simulink model "general_pi_model"  (R2024b)
settings: Solver=VariableStepAuto  StartTime=0.0  StopTime=t_stop  RelTol=1e-3
values from neighbouring files (symbols this model uses):
  C = 1.97e3/2    (= 985)    [general_pi_init.m]
  L = 5.21e-5    (= 5.21e-05)    [general_pi_init.m]
  SIL = sqrt(L/C)    [general_pi_init.m]
libraries: fl_lib x128, nesl_utility x81, ee_lib x1
(part 1 of 3)
settings Model: Creator=inyongkim  LastModifiedBy=inyongkim

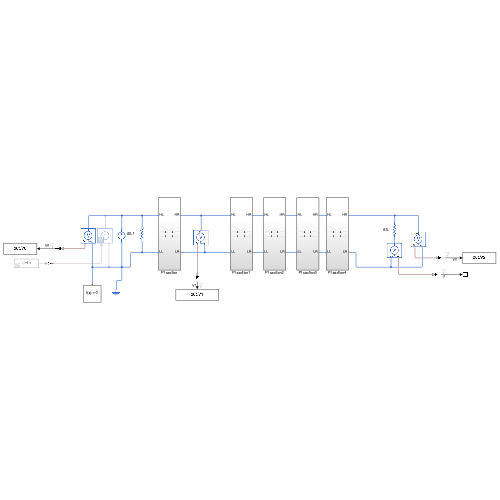
[thumbnail: Simulink's stored preview of the top-level diagram]
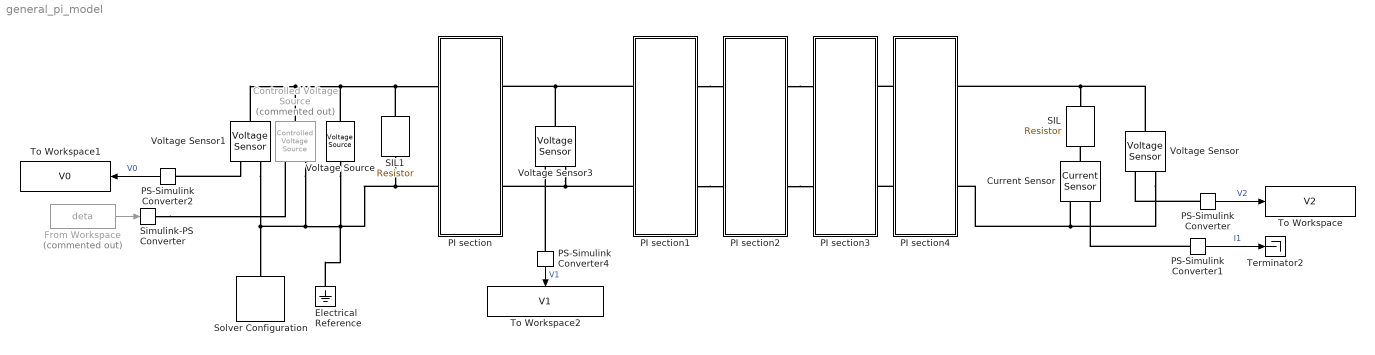
== system general_pi_model ==
  Controlled Voltage Source : fl_lib/Electrical/Electrical Sources/Controlled Voltage Source  Commented=on
  Current Sensor : fl_lib/Electrical/Electrical Sensors/Current Sensor
  Electrical Reference : fl_lib/Electrical/Electrical Elements/Electrical Reference
  From Workspace : FromWorkspace  Commented=on  VariableName=deta
  PI section : Subsystem
  PI section1 : Subsystem
  PI section2 : Subsystem
  PI section3 : Subsystem
  PI section4 : Subsystem
  PS-Simulink Converter{,1..2,4} (4 alike) : nesl_utility/PS-Simulink Converter  PhysicalDomain=network_engine_domain  SubClassName=ps_output  LeftPortType=input  RightPortType=output  PseudoPeriodic=off  Frequencies=[]  VectorFormat=inherit  Unit=inherit  AffineConversion=off
  SIL : fl_lib/Electrical/Electrical Elements/Resistor  R=SIL Ohm  i_specify=off  i_priority=None  i=0 A  i_nominal_specify=off  i_nominal_value=1  i_nominal_unit=A  v_specify=off  v_priority=None  v=0 V  v_nominal_specify=off  v_nominal_value=1  v_nominal_unit=V
  SIL1 : fl_lib/Electrical/Electrical Elements/Resistor  R=SIL*1e12 Ohm  i_specify=off  i_priority=None  i=0 A  i_nominal_specify=off  i_nominal_value=1  i_nominal_unit=A  v_specify=off  v_priority=None  v=0 V  v_nominal_specify=off  v_nominal_value=1  v_nominal_unit=V
  Simulink-PS Converter : nesl_utility/Simulink-PS Converter  PhysicalDomain=network_engine_domain  SubClassName=ps_input  LeftPortType=input  RightPortType=output  PseudoPeriodic=off  Frequencies=[]  NoiseDistribution=none  NoiseParameters=[]  Unit=V  AffineConversion=off  FilteringAndDerivatives=provide  SimscapeFilterOrder=1  InputFilterTimeConstant=0.001  UdotUserProvided=0
  Solver Configuration : nesl_utility/Solver Configuration  PhysicalDomain=network_engine_domain  SubClassName=solver  LeftPortType=input  RightPortType=generic  Tones=[]  Harmonics=[]  SimulateNoise=off  Profile=off  UseLocalSampling=off  EnableSwitchedLinearOptims=on  FrequencyDomain=off  UseCCode=off  RelTol=0.001  AbsTol=0.001  MinStep=1e-09  ToWorkspace=off  RevertToSquareIcSolve=off  NumHomotopyIterations=100  PhasorMode=off  PhasorModeNumHarmonics=1  ConsistencySolver=NEWTON_XTOL_AFTER_FTOL  IndexReductionMethod=DerivativeReplacement  DoDC=off  ResidualTolerance=1e-09  ConsistencyTolSource=GLOBAL  ConsistencyAbsTol=0.001  ConsistencyRelTol=0.001  ConsistencyTolFactor=0.001  UseLocalSolver=off  LocalSolverChoice=NE_BACKWARD_EULER_ADVANCER  ResolveIndetEquations=on  FunctionEvalNumThread=1  LocalSolverSampleTime=0.001  DoFixedCost=off  MaxNonlinIter=3  MaxModeIter=2  ComputeImpulses=off  ImpulseIterations=2  LinearAlgebra=auto  LinearAlgebraNumThread=0  EquationFormulation=NE_TIME_EF  DelaysMemoryBudget=1024  AutomaticFiltering=on  FilteringTimeConstant=0.001  PartitionStorageMethod=AS_NEEDED  PartitionMemoryBudget=1024  PartitionMethod=ROBUST  MultibodyUseLocalSolver=off  MultibodyLocalSolverChoice=ODE1  MultibodyLocalSolverSampleTime=0.001
  Terminator2 : Terminator
  To Workspace : ToWorkspace  VariableName=V2  SaveFormat=Timeseries  SampleTime=-1
  To Workspace1 : ToWorkspace  VariableName=V0  SaveFormat=Timeseries  SampleTime=-1
  To Workspace2 : ToWorkspace  VariableName=V1  SaveFormat=Timeseries  SampleTime=-1
  Voltage Sensor : fl_lib/Electrical/Electrical Sensors/Voltage Sensor
  Voltage Sensor1 : fl_lib/Electrical/Electrical Sensors/Voltage Sensor
  Voltage Sensor3 : fl_lib/Electrical/Electrical Sensors/Voltage Sensor
  Voltage Source : ee_lib/Sources/Voltage Source  dc_voltage=0 V  ac_voltage=1 V  ac_shift=0 rad  ac_frequency=0.1 Hz  noise_mode=ee.enum.sources.noise.Disabled  PSD=0 V^2/Hz  sample_time=1e-3 s  repeatability=ee.enum.sources.repeatability.NotRepeatable  user_seed=0  auto_seed=3499211588  i_specify=off  i_priority=None  i=0 A  i_nominal_specify=off  i_nominal_value=1  i_nominal_unit=A  v_specify=off  v_priority=None  v=0 V  v_nominal_specify=off  v_nominal_value=1  v_nominal_unit=V
  wires:
  PS-Simulink Converter/1 -> To Workspace/1  "V2"
  PS-Simulink Converter1/1 -> Terminator2/1  "I1"
  PS-Simulink Converter2/1 -> To Workspace1/1  "V0"
  From Workspace/1 -> Simulink-PS Converter/1
  PS-Simulink Converter4/1 -> To Workspace2/1  "V1"
  connections:
  Voltage Source/RConn1 -- Controlled Voltage Source/RConn2 -- Solver Configuration/RConn1 -- Voltage Sensor1/RConn2 -- SIL1/RConn1 -- PI section/LConn2 -- Electrical Reference/LConn1
  Voltage Sensor1/LConn1 -- SIL1/LConn1 -- PI section/LConn1 -- Voltage Source/LConn1 -- Controlled Voltage Source/LConn1
  Voltage Sensor/LConn1 -- PI section4/RConn1 -- SIL/LConn1
  PS-Simulink Converter/LConn1 -- Voltage Sensor/RConn1
  Current Sensor/LConn1 -- SIL/RConn1
  PS-Simulink Converter1/LConn1 -- Current Sensor/RConn1
  Voltage Sensor1/RConn1 -- PS-Simulink Converter2/LConn1
  Simulink-PS Converter/RConn1 -- Controlled Voltage Source/RConn1
  PS-Simulink Converter4/LConn1 -- Voltage Sensor3/RConn1
  Voltage Sensor3/LConn1 -- PI section1/LConn1 -- PI section/RConn1
  Voltage Sensor3/RConn2 -- PI section/RConn2 -- PI section1/LConn2
  Voltage Sensor/RConn2 -- PI section4/RConn2 -- Current Sensor/RConn2
  PI section1/RConn1 -- PI section2/LConn1
  PI section1/RConn2 -- PI section2/LConn2
  PI section2/RConn1 -- PI section3/LConn1
  PI section2/RConn2 -- PI section3/LConn2
  PI section4/LConn1 -- PI section3/RConn1
  PI section4/LConn2 -- PI section3/RConn2

== system general_pi_model/PI section ==
  General C : Subsystem
      settings: PortSchema="{\"entries\":[{\"content\":{\"sides\":[{\"content\":{},\"type\":\"ConnectorPlacement.EquallySpacedRectSide\",\"uuid\":\"54c7c027-76dd-4589-a14d-62021aaba10d\"},{\"content\":{\"side\":\"RIGHT\"},\"type\":\"ConnectorPlacement.EquallySpacedRectSide\",\"uuid\":\"5fae45fc-fbd0-44d0-9d3d-94b3e56c48e3\"},{\"content\":{\"connectorIds\":[\"LConn1\"],\"side\":\"TOP\"},\"type\":\"ConnectorPlacement.EquallySpacedRectSide\",\"uuid\":\"b6847d7e-9825-46ad-84aa-5df9156d119d\"},{\"content\":{\"connectorIds\":[\"RConn1\"],\"side\":\"BOTTOM\"},\"type\":\"ConnectorPlacement.EquallySpacedRectSide\",\"uuid\":\"1394d42d-8985-4309-a3e0-31ed6b8c9496\"}]},\"type\":\"ConnectorPlacement.EquallySpacedConnector\",\"uuid\":\"6a4af355-2598-47af-9220-e6e09375ad72\"}],\"packageUris\":[\"http://schema.mathworks.com/mf0/Connector/R2020b\"],\"version\":\"1.0\"}"
  General C1 : Subsystem
      settings: PortSchema="{\"entries\":[{\"content\":{\"sides\":[{\"content\":{},\"type\":\"ConnectorPlacement.EquallySpacedRectSide\",\"uuid\":\"54c7c027-76dd-4589-a14d-62021aaba10d\"},{\"content\":{\"side\":\"RIGHT\"},\"type\":\"ConnectorPlacement.EquallySpacedRectSide\",\"uuid\":\"5fae45fc-fbd0-44d0-9d3d-94b3e56c48e3\"},{\"content\":{\"connectorIds\":[\"LConn1\"],\"side\":\"TOP\"},\"type\":\"ConnectorPlacement.EquallySpacedRectSide\",\"uuid\":\"b6847d7e-9825-46ad-84aa-5df9156d119d\"},{\"content\":{\"connectorIds\":[\"RConn1\"],\"side\":\"BOTTOM\"},\"type\":\"ConnectorPlacement.EquallySpacedRectSide\",\"uuid\":\"1394d42d-8985-4309-a3e0-31ed6b8c9496\"}]},\"type\":\"ConnectorPlacement.EquallySpacedConnector\",\"uuid\":\"6a4af355-2598-47af-9220-e6e09375ad72\"}],\"packageUris\":[\"http://schema.mathworks.com/mf0/Connector/R2020b\"],\"version\":\"1.0\"}"
  General L : Subsystem
      settings: PortSchema="{\"entries\":[{\"content\":{\"sides\":[{\"content\":{},\"type\":\"ConnectorPlacement.EquallySpacedRectSide\",\"uuid\":\"54c7c027-76dd-4589-a14d-62021aaba10d\"},{\"content\":{\"side\":\"RIGHT\"},\"type\":\"ConnectorPlacement.EquallySpacedRectSide\",\"uuid\":\"5fae45fc-fbd0-44d0-9d3d-94b3e56c48e3\"},{\"content\":{\"connectorIds\":[\"LConn1\"],\"side\":\"TOP\"},\"type\":\"ConnectorPlacement.EquallySpacedRectSide\",\"uuid\":\"b6847d7e-9825-46ad-84aa-5df9156d119d\"},{\"content\":{\"connectorIds\":[\"RConn1\"],\"side\":\"BOTTOM\"},\"type\":\"ConnectorPlacement.EquallySpacedRectSide\",\"uuid\":\"7b301271-0a77-4acb-8843-591cb23b0585\"}]},\"type\":\"ConnectorPlacement.EquallySpacedConnector\",\"uuid\":\"6a4af355-2598-47af-9220-e6e09375ad72\"}],\"packageUris\":[\"http://schema.mathworks.com/mf0/Connector/R2020b\"],\"version\":\"1.0\"}"
  HL : PMIOPort  Side=Left
  HR : PMIOPort  Port=2  Side=Right
  LL : PMIOPort  Port=3  Side=Left
  LR : PMIOPort  Port=4  Side=Right
  connections:
  General L/RConn1 -- HR/RConn1 -- General C1/LConn1
  General C1/RConn1 -- General C/RConn1 -- LL/RConn1 -- LR/RConn1
  General C/LConn1 -- HL/RConn1 -- General L/LConn1

== system general_pi_model/PI section1 ==
  General C : Subsystem
      settings: PortSchema="{\"entries\":[{\"content\":{\"sides\":[{\"content\":{},\"type\":\"ConnectorPlacement.EquallySpacedRectSide\",\"uuid\":\"54c7c027-76dd-4589-a14d-62021aaba10d\"},{\"content\":{\"side\":\"RIGHT\"},\"type\":\"ConnectorPlacement.EquallySpacedRectSide\",\"uuid\":\"5fae45fc-fbd0-44d0-9d3d-94b3e56c48e3\"},{\"content\":{\"connectorIds\":[\"LConn1\"],\"side\":\"TOP\"},\"type\":\"ConnectorPlacement.EquallySpacedRectSide\",\"uuid\":\"b6847d7e-9825-46ad-84aa-5df9156d119d\"},{\"content\":{\"connectorIds\":[\"RConn1\"],\"side\":\"BOTTOM\"},\"type\":\"ConnectorPlacement.EquallySpacedRectSide\",\"uuid\":\"1394d42d-8985-4309-a3e0-31ed6b8c9496\"}]},\"type\":\"ConnectorPlacement.EquallySpacedConnector\",\"uuid\":\"6a4af355-2598-47af-9220-e6e09375ad72\"}],\"packageUris\":[\"http://schema.mathworks.com/mf0/Connector/R2020b\"],\"version\":\"1.0\"}"
  General C1 : Subsystem
      settings: PortSchema="{\"entries\":[{\"content\":{\"sides\":[{\"content\":{},\"type\":\"ConnectorPlacement.EquallySpacedRectSide\",\"uuid\":\"54c7c027-76dd-4589-a14d-62021aaba10d\"},{\"content\":{\"side\":\"RIGHT\"},\"type\":\"ConnectorPlacement.EquallySpacedRectSide\",\"uuid\":\"5fae45fc-fbd0-44d0-9d3d-94b3e56c48e3\"},{\"content\":{\"connectorIds\":[\"LConn1\"],\"side\":\"TOP\"},\"type\":\"ConnectorPlacement.EquallySpacedRectSide\",\"uuid\":\"b6847d7e-9825-46ad-84aa-5df9156d119d\"},{\"content\":{\"connectorIds\":[\"RConn1\"],\"side\":\"BOTTOM\"},\"type\":\"ConnectorPlacement.EquallySpacedRectSide\",\"uuid\":\"1394d42d-8985-4309-a3e0-31ed6b8c9496\"}]},\"type\":\"ConnectorPlacement.EquallySpacedConnector\",\"uuid\":\"6a4af355-2598-47af-9220-e6e09375ad72\"}],\"packageUris\":[\"http://schema.mathworks.com/mf0/Connector/R2020b\"],\"version\":\"1.0\"}"
  General L : Subsystem
      settings: PortSchema="{\"entries\":[{\"content\":{\"sides\":[{\"content\":{},\"type\":\"ConnectorPlacement.EquallySpacedRectSide\",\"uuid\":\"54c7c027-76dd-4589-a14d-62021aaba10d\"},{\"content\":{\"side\":\"RIGHT\"},\"type\":\"ConnectorPlacement.EquallySpacedRectSide\",\"uuid\":\"5fae45fc-fbd0-44d0-9d3d-94b3e56c48e3\"},{\"content\":{\"connectorIds\":[\"LConn1\"],\"side\":\"TOP\"},\"type\":\"ConnectorPlacement.EquallySpacedRectSide\",\"uuid\":\"b6847d7e-9825-46ad-84aa-5df9156d119d\"},{\"content\":{\"connectorIds\":[\"RConn1\"],\"side\":\"BOTTOM\"},\"type\":\"ConnectorPlacement.EquallySpacedRectSide\",\"uuid\":\"7b301271-0a77-4acb-8843-591cb23b0585\"}]},\"type\":\"ConnectorPlacement.EquallySpacedConnector\",\"uuid\":\"6a4af355-2598-47af-9220-e6e09375ad72\"}],\"packageUris\":[\"http://schema.mathworks.com/mf0/Connector/R2020b\"],\"version\":\"1.0\"}"
  HL : PMIOPort  Side=Left
  HR : PMIOPort  Port=2  Side=Right
  LL : PMIOPort  Port=3  Side=Left
  LR : PMIOPort  Port=4  Side=Right
  connections:
  General L/RConn1 -- General C1/LConn1 -- HR/RConn1
  LR/RConn1 -- General C1/RConn1 -- LL/RConn1 -- General C/RConn1
  General C/LConn1 -- General L/LConn1 -- HL/RConn1

== system general_pi_model/PI section2 ==
  General C : Subsystem
      settings: PortSchema="{\"entries\":[{\"content\":{\"sides\":[{\"content\":{},\"type\":\"ConnectorPlacement.EquallySpacedRectSide\",\"uuid\":\"54c7c027-76dd-4589-a14d-62021aaba10d\"},{\"content\":{\"side\":\"RIGHT\"},\"type\":\"ConnectorPlacement.EquallySpacedRectSide\",\"uuid\":\"5fae45fc-fbd0-44d0-9d3d-94b3e56c48e3\"},{\"content\":{\"connectorIds\":[\"LConn1\"],\"side\":\"TOP\"},\"type\":\"ConnectorPlacement.EquallySpacedRectSide\",\"uuid\":\"b6847d7e-9825-46ad-84aa-5df9156d119d\"},{\"content\":{\"connectorIds\":[\"RConn1\"],\"side\":\"BOTTOM\"},\"type\":\"ConnectorPlacement.EquallySpacedRectSide\",\"uuid\":\"1394d42d-8985-4309-a3e0-31ed6b8c9496\"}]},\"type\":\"ConnectorPlacement.EquallySpacedConnector\",\"uuid\":\"6a4af355-2598-47af-9220-e6e09375ad72\"}],\"packageUris\":[\"http://schema.mathworks.com/mf0/Connector/R2020b\"],\"version\":\"1.0\"}"
  General C1 : Subsystem
      settings: PortSchema="{\"entries\":[{\"content\":{\"sides\":[{\"content\":{},\"type\":\"ConnectorPlacement.EquallySpacedRectSide\",\"uuid\":\"54c7c027-76dd-4589-a14d-62021aaba10d\"},{\"content\":{\"side\":\"RIGHT\"},\"type\":\"ConnectorPlacement.EquallySpacedRectSide\",\"uuid\":\"5fae45fc-fbd0-44d0-9d3d-94b3e56c48e3\"},{\"content\":{\"connectorIds\":[\"LConn1\"],\"side\":\"TOP\"},\"type\":\"ConnectorPlacement.EquallySpacedRectSide\",\"uuid\":\"b6847d7e-9825-46ad-84aa-5df9156d119d\"},{\"content\":{\"connectorIds\":[\"RConn1\"],\"side\":\"BOTTOM\"},\"type\":\"ConnectorPlacement.EquallySpacedRectSide\",\"uuid\":\"1394d42d-8985-4309-a3e0-31ed6b8c9496\"}]},\"type\":\"ConnectorPlacement.EquallySpacedConnector\",\"uuid\":\"6a4af355-2598-47af-9220-e6e09375ad72\"}],\"packageUris\":[\"http://schema.mathworks.com/mf0/Connector/R2020b\"],\"version\":\"1.0\"}"
  General L : Subsystem
      settings: PortSchema="{\"entries\":[{\"content\":{\"sides\":[{\"content\":{},\"type\":\"ConnectorPlacement.EquallySpacedRectSide\",\"uuid\":\"54c7c027-76dd-4589-a14d-62021aaba10d\"},{\"content\":{\"side\":\"RIGHT\"},\"type\":\"ConnectorPlacement.EquallySpacedRectSide\",\"uuid\":\"5fae45fc-fbd0-44d0-9d3d-94b3e56c48e3\"},{\"content\":{\"connectorIds\":[\"LConn1\"],\"side\":\"TOP\"},\"type\":\"ConnectorPlacement.EquallySpacedRectSide\",\"uuid\":\"b6847d7e-9825-46ad-84aa-5df9156d119d\"},{\"content\":{\"connectorIds\":[\"RConn1\"],\"side\":\"BOTTOM\"},\"type\":\"ConnectorPlacement.EquallySpacedRectSide\",\"uuid\":\"7b301271-0a77-4acb-8843-591cb23b0585\"}]},\"type\":\"ConnectorPlacement.EquallySpacedConnector\",\"uuid\":\"6a4af355-2598-47af-9220-e6e09375ad72\"}],\"packageUris\":[\"http://schema.mathworks.com/mf0/Connector/R2020b\"],\"version\":\"1.0\"}"
  HL : PMIOPort  Side=Left
  HR : PMIOPort  Port=2  Side=Right
  LL : PMIOPort  Port=3  Side=Left
  LR : PMIOPort  Port=4  Side=Right
  connections:
  General L/RConn1 -- General C1/LConn1 -- HR/RConn1
  LR/RConn1 -- General C1/RConn1 -- LL/RConn1 -- General C/RConn1
  General C/LConn1 -- General L/LConn1 -- HL/RConn1

== system general_pi_model/PI section3 ==
  General C : Subsystem
      settings: PortSchema="{\"entries\":[{\"content\":{\"sides\":[{\"content\":{},\"type\":\"ConnectorPlacement.EquallySpacedRectSide\",\"uuid\":\"54c7c027-76dd-4589-a14d-62021aaba10d\"},{\"content\":{\"side\":\"RIGHT\"},\"type\":\"ConnectorPlacement.EquallySpacedRectSide\",\"uuid\":\"5fae45fc-fbd0-44d0-9d3d-94b3e56c48e3\"},{\"content\":{\"connectorIds\":[\"LConn1\"],\"side\":\"TOP\"},\"type\":\"ConnectorPlacement.EquallySpacedRectSide\",\"uuid\":\"b6847d7e-9825-46ad-84aa-5df9156d119d\"},{\"content\":{\"connectorIds\":[\"RConn1\"],\"side\":\"BOTTOM\"},\"type\":\"ConnectorPlacement.EquallySpacedRectSide\",\"uuid\":\"1394d42d-8985-4309-a3e0-31ed6b8c9496\"}]},\"type\":\"ConnectorPlacement.EquallySpacedConnector\",\"uuid\":\"6a4af355-2598-47af-9220-e6e09375ad72\"}],\"packageUris\":[\"http://schema.mathworks.com/mf0/Connector/R2020b\"],\"version\":\"1.0\"}"
  General C1 : Subsystem
      settings: PortSchema="{\"entries\":[{\"content\":{\"sides\":[{\"content\":{},\"type\":\"ConnectorPlacement.EquallySpacedRectSide\",\"uuid\":\"54c7c027-76dd-4589-a14d-62021aaba10d\"},{\"content\":{\"side\":\"RIGHT\"},\"type\":\"ConnectorPlacement.EquallySpacedRectSide\",\"uuid\":\"5fae45fc-fbd0-44d0-9d3d-94b3e56c48e3\"},{\"content\":{\"connectorIds\":[\"LConn1\"],\"side\":\"TOP\"},\"type\":\"ConnectorPlacement.EquallySpacedRectSide\",\"uuid\":\"b6847d7e-9825-46ad-84aa-5df9156d119d\"},{\"content\":{\"connectorIds\":[\"RConn1\"],\"side\":\"BOTTOM\"},\"type\":\"ConnectorPlacement.EquallySpacedRectSide\",\"uuid\":\"1394d42d-8985-4309-a3e0-31ed6b8c9496\"}]},\"type\":\"ConnectorPlacement.EquallySpacedConnector\",\"uuid\":\"6a4af355-2598-47af-9220-e6e09375ad72\"}],\"packageUris\":[\"http://schema.mathworks.com/mf0/Connector/R2020b\"],\"version\":\"1.0\"}"
  General L : Subsystem
      settings: PortSchema="{\"entries\":[{\"content\":{\"sides\":[{\"content\":{},\"type\":\"ConnectorPlacement.EquallySpacedRectSide\",\"uuid\":\"54c7c027-76dd-4589-a14d-62021aaba10d\"},{\"content\":{\"side\":\"RIGHT\"},\"type\":\"ConnectorPlacement.EquallySpacedRectSide\",\"uuid\":\"5fae45fc-fbd0-44d0-9d3d-94b3e56c48e3\"},{\"content\":{\"connectorIds\":[\"LConn1\"],\"side\":\"TOP\"},\"type\":\"ConnectorPlacement.EquallySpacedRectSide\",\"uuid\":\"b6847d7e-9825-46ad-84aa-5df9156d119d\"},{\"content\":{\"connectorIds\":[\"RConn1\"],\"side\":\"BOTTOM\"},\"type\":\"ConnectorPlacement.EquallySpacedRectSide\",\"uuid\":\"7b301271-0a77-4acb-8843-591cb23b0585\"}]},\"type\":\"ConnectorPlacement.EquallySpacedConnector\",\"uuid\":\"6a4af355-2598-47af-9220-e6e09375ad72\"}],\"packageUris\":[\"http://schema.mathworks.com/mf0/Connector/R2020b\"],\"version\":\"1.0\"}"
  HL : PMIOPort  Side=Left
  HR : PMIOPort  Port=2  Side=Right
  LL : PMIOPort  Port=3  Side=Left
  LR : PMIOPort  Port=4  Side=Right
  connections:
  General L/RConn1 -- General C1/LConn1 -- HR/RConn1
  LR/RConn1 -- General C1/RConn1 -- LL/RConn1 -- General C/RConn1
  General C/LConn1 -- General L/LConn1 -- HL/RConn1

== system general_pi_model/PI section4 ==
  General C : Subsystem
      settings: PortSchema="{\"entries\":[{\"content\":{\"sides\":[{\"content\":{},\"type\":\"ConnectorPlacement.EquallySpacedRectSide\",\"uuid\":\"54c7c027-76dd-4589-a14d-62021aaba10d\"},{\"content\":{\"side\":\"RIGHT\"},\"type\":\"ConnectorPlacement.EquallySpacedRectSide\",\"uuid\":\"5fae45fc-fbd0-44d0-9d3d-94b3e56c48e3\"},{\"content\":{\"connectorIds\":[\"LConn1\"],\"side\":\"TOP\"},\"type\":\"ConnectorPlacement.EquallySpacedRectSide\",\"uuid\":\"b6847d7e-9825-46ad-84aa-5df9156d119d\"},{\"content\":{\"connectorIds\":[\"RConn1\"],\"side\":\"BOTTOM\"},\"type\":\"ConnectorPlacement.EquallySpacedRectSide\",\"uuid\":\"1394d42d-8985-4309-a3e0-31ed6b8c9496\"}]},\"type\":\"ConnectorPlacement.EquallySpacedConnector\",\"uuid\":\"6a4af355-2598-47af-9220-e6e09375ad72\"}],\"packageUris\":[\"http://schema.mathworks.com/mf0/Connector/R2020b\"],\"version\":\"1.0\"}"
  General C1 : Subsystem
      settings: PortSchema="{\"entries\":[{\"content\":{\"sides\":[{\"content\":{},\"type\":\"ConnectorPlacement.EquallySpacedRectSide\",\"uuid\":\"54c7c027-76dd-4589-a14d-62021aaba10d\"},{\"content\":{\"side\":\"RIGHT\"},\"type\":\"ConnectorPlacement.EquallySpacedRectSide\",\"uuid\":\"5fae45fc-fbd0-44d0-9d3d-94b3e56c48e3\"},{\"content\":{\"connectorIds\":[\"LConn1\"],\"side\":\"TOP\"},\"type\":\"ConnectorPlacement.EquallySpacedRectSide\",\"uuid\":\"b6847d7e-9825-46ad-84aa-5df9156d119d\"},{\"content\":{\"connectorIds\":[\"RConn1\"],\"side\":\"BOTTOM\"},\"type\":\"ConnectorPlacement.EquallySpacedRectSide\",\"uuid\":\"1394d42d-8985-4309-a3e0-31ed6b8c9496\"}]},\"type\":\"ConnectorPlacement.EquallySpacedConnector\",\"uuid\":\"6a4af355-2598-47af-9220-e6e09375ad72\"}],\"packageUris\":[\"http://schema.mathworks.com/mf0/Connector/R2020b\"],\"version\":\"1.0\"}"
  General L : Subsystem
      settings: PortSchema="{\"entries\":[{\"content\":{\"sides\":[{\"content\":{},\"type\":\"ConnectorPlacement.EquallySpacedRectSide\",\"uuid\":\"54c7c027-76dd-4589-a14d-62021aaba10d\"},{\"content\":{\"side\":\"RIGHT\"},\"type\":\"ConnectorPlacement.EquallySpacedRectSide\",\"uuid\":\"5fae45fc-fbd0-44d0-9d3d-94b3e56c48e3\"},{\"content\":{\"connectorIds\":[\"LConn1\"],\"side\":\"TOP\"},\"type\":\"ConnectorPlacement.EquallySpacedRectSide\",\"uuid\":\"b6847d7e-9825-46ad-84aa-5df9156d119d\"},{\"content\":{\"connectorIds\":[\"RConn1\"],\"side\":\"BOTTOM\"},\"type\":\"ConnectorPlacement.EquallySpacedRectSide\",\"uuid\":\"7b301271-0a77-4acb-8843-591cb23b0585\"}]},\"type\":\"ConnectorPlacement.EquallySpacedConnector\",\"uuid\":\"6a4af355-2598-47af-9220-e6e09375ad72\"}],\"packageUris\":[\"http://schema.mathworks.com/mf0/Connector/R2020b\"],\"version\":\"1.0\"}"
  HL : PMIOPort  Side=Left
  HR : PMIOPort  Port=2  Side=Right
  LL : PMIOPort  Port=3  Side=Left
  LR : PMIOPort  Port=4  Side=Right
  connections:
  General L/RConn1 -- General C1/LConn1 -- HR/RConn1
  LR/RConn1 -- General C1/RConn1 -- LL/RConn1 -- General C/RConn1
  General C/LConn1 -- General L/LConn1 -- HL/RConn1

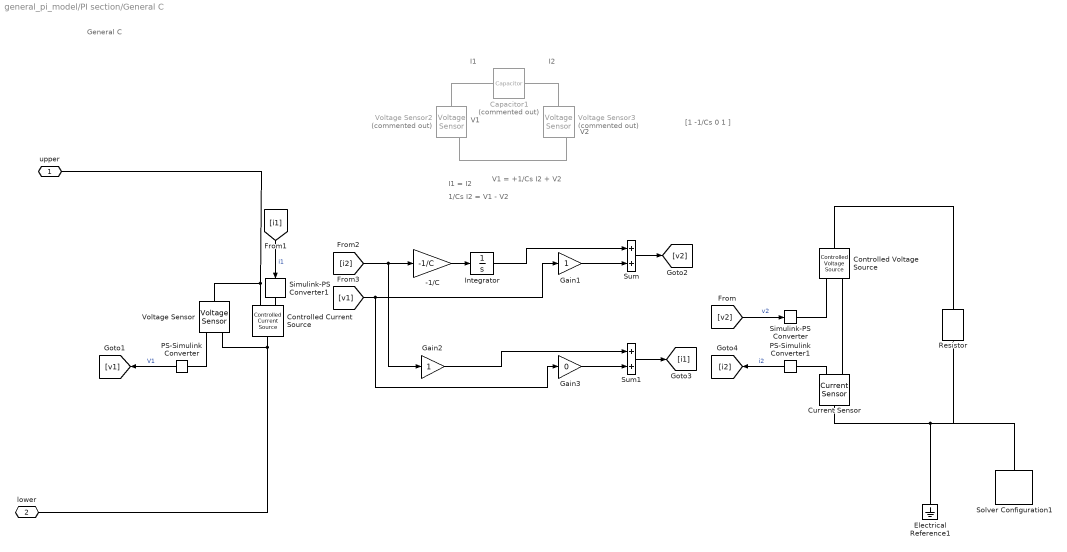
== system general_pi_model/PI section/General C ==
  note: General C
  note: V1
  note: V1 = +1/Cs I2 + V2
  note: I2
  note: I1 = I2
  note: 1/Cs I2 = V1 - V2
  note: V2
  note: [1 -1/Cs
      | 0 1 ]
  note: I1
  -1/C : Gain  Gain=-1/C
  Capacitor1 : fl_lib/Electrical/Electrical Elements/Capacitor  Commented=on  c=1e-6 F  r=1e-6 Ohm  g=0 1/Ohm  i_specify=off  i_priority=None  i=0 A  i_nominal_specify=off  i_nominal_value=1  i_nominal_unit=A  v_specify=off  v_priority=None  v=0 V  v_nominal_specify=off  v_nominal_value=1  v_nominal_unit=V  vc_specify=off  vc_priority=High  vc=0 V  vc_nominal_specify=off  vc_nominal_value=1  vc_nominal_unit=V
  Controlled Current Source : fl_lib/Electrical/Electrical Sources/Controlled Current Source
  Controlled Voltage Source : fl_lib/Electrical/Electrical Sources/Controlled Voltage Source
  Current Sensor : fl_lib/Electrical/Electrical Sensors/Current Sensor
  Electrical Reference1 : fl_lib/Electrical/Electrical Elements/Electrical Reference
  Gain1 : Gain
  Gain2 : Gain
  Gain3 : Gain  Gain=0
  Integrator : Integrator
  PS-Simulink Converter : nesl_utility/PS-Simulink Converter  PhysicalDomain=network_engine_domain  SubClassName=ps_output  LeftPortType=input  RightPortType=output  PseudoPeriodic=off  Frequencies=[]  VectorFormat=inherit  Unit=inherit  AffineConversion=off
  PS-Simulink Converter1 : nesl_utility/PS-Simulink Converter  PhysicalDomain=network_engine_domain  SubClassName=ps_output  LeftPortType=input  RightPortType=output  PseudoPeriodic=off  Frequencies=[]  VectorFormat=inherit  Unit=inherit  AffineConversion=off
  Resistor : fl_lib/Electrical/Electrical Elements/Resistor  R=1e-12 Ohm  i_specify=off  i_priority=None  i=0 A  i_nominal_specify=off  i_nominal_value=1  i_nominal_unit=A  v_specify=off  v_priority=None  v=0 V  v_nominal_specify=off  v_nominal_value=1  v_nominal_unit=V
  Simulink-PS Converter : nesl_utility/Simulink-PS Converter  PhysicalDomain=network_engine_domain  SubClassName=ps_input  LeftPortType=input  RightPortType=output  PseudoPeriodic=off  Frequencies=[]  NoiseDistribution=none  NoiseParameters=[]  Unit=V  AffineConversion=off  FilteringAndDerivatives=provide  SimscapeFilterOrder=1  InputFilterTimeConstant=0.001  UdotUserProvided=0
  Simulink-PS Converter1 : nesl_utility/Simulink-PS Converter  PhysicalDomain=network_engine_domain  SubClassName=ps_input  LeftPortType=input  RightPortType=output  PseudoPeriodic=off  Frequencies=[]  NoiseDistribution=none  NoiseParameters=[]  Unit=A  AffineConversion=off  FilteringAndDerivatives=provide  SimscapeFilterOrder=1  InputFilterTimeConstant=0.001  UdotUserProvided=0
  Solver Configuration1 : nesl_utility/Solver Configuration  PhysicalDomain=network_engine_domain  SubClassName=solver  LeftPortType=input  RightPortType=generic  Tones=[]  Harmonics=[]  SimulateNoise=off  Profile=off  UseLocalSampling=off  EnableSwitchedLinearOptims=on  FrequencyDomain=off  UseCCode=off  RelTol=0.001  AbsTol=0.001  MinStep=1e-09  ToWorkspace=off  RevertToSquareIcSolve=off  NumHomotopyIterations=100  PhasorMode=off  PhasorModeNumHarmonics=1  ConsistencySolver=NEWTON_XTOL_AFTER_FTOL  IndexReductionMethod=DerivativeReplacement  DoDC=off  ResidualTolerance=1e-09  ConsistencyTolSource=GLOBAL  ConsistencyAbsTol=0.001  ConsistencyRelTol=0.001  ConsistencyTolFactor=0.001  UseLocalSolver=off  LocalSolverChoice=NE_BACKWARD_EULER_ADVANCER  ResolveIndetEquations=on  FunctionEvalNumThread=1  LocalSolverSampleTime=0.001  DoFixedCost=off  MaxNonlinIter=3  MaxModeIter=2  ComputeImpulses=off  ImpulseIterations=2  LinearAlgebra=auto  LinearAlgebraNumThread=0  EquationFormulation=NE_TIME_EF  DelaysMemoryBudget=1024  AutomaticFiltering=on  FilteringTimeConstant=0.001  PartitionStorageMethod=AS_NEEDED  PartitionMemoryBudget=1024  PartitionMethod=ROBUST  MultibodyUseLocalSolver=off  MultibodyLocalSolverChoice=ODE1  MultibodyLocalSolverSampleTime=0.001
  Sum : Sum
  Sum1 : Sum
  Voltage Sensor : fl_lib/Electrical/Electrical Sensors/Voltage Sensor
  Voltage Sensor2 : fl_lib/Electrical/Electrical Sensors/Voltage Sensor  Commented=on
  Voltage Sensor3 : fl_lib/Electrical/Electrical Sensors/Voltage Sensor  Commented=on
  upper : PMIOPort  Side=Left
  lower : PMIOPort  Port=2  Side=Right
  wires:
  Sum1/1 -> [i1]
  Sum/1 -> [v2]
  [i2] -> Gain2/1, -1/C/1
  [v1] -> Gain1/1, Gain3/1
  Gain2/1 -> Sum1/1
  Gain3/1 -> Sum1/2
  Integrator/1 -> Sum/1
  Gain1/1 -> Sum/2
  -1/C/1 -> Integrator/1
  [i1] -> Simulink-PS Converter1/1  "i1"
  PS-Simulink Converter/1 -> [v1]  "V1"
  [v2] -> Simulink-PS Converter/1  "v2"
  PS-Simulink Converter1/1 -> [i2]  "i2"
  connections:
  Controlled Current Source/LConn1 -- lower/RConn1 -- Voltage Sensor/RConn2
  Voltage Sensor3/RConn2 -- Voltage Sensor2/RConn2
  Voltage Sensor3/LConn1 -- Capacitor1/RConn1
  Voltage Sensor2/LConn1 -- Capacitor1/LConn1
  Electrical Reference1/LConn1 -- Solver Configuration1/RConn1 -- Resistor/RConn1 -- Current Sensor/LConn1
  Resistor/LConn1 -- Controlled Voltage Source/LConn1
  Simulink-PS Converter/RConn1 -- Controlled Voltage Source/RConn1
  PS-Simulink Converter1/LConn1 -- Current Sensor/RConn1
  Voltage Sensor/RConn1 -- PS-Simulink Converter/LConn1
  Current Sensor/RConn2 -- Controlled Voltage Source/RConn2
  Controlled Current Source/RConn1 -- Simulink-PS Converter1/RConn1
  Controlled Current Source/RConn2 -- upper/RConn1 -- Voltage Sensor/LConn1

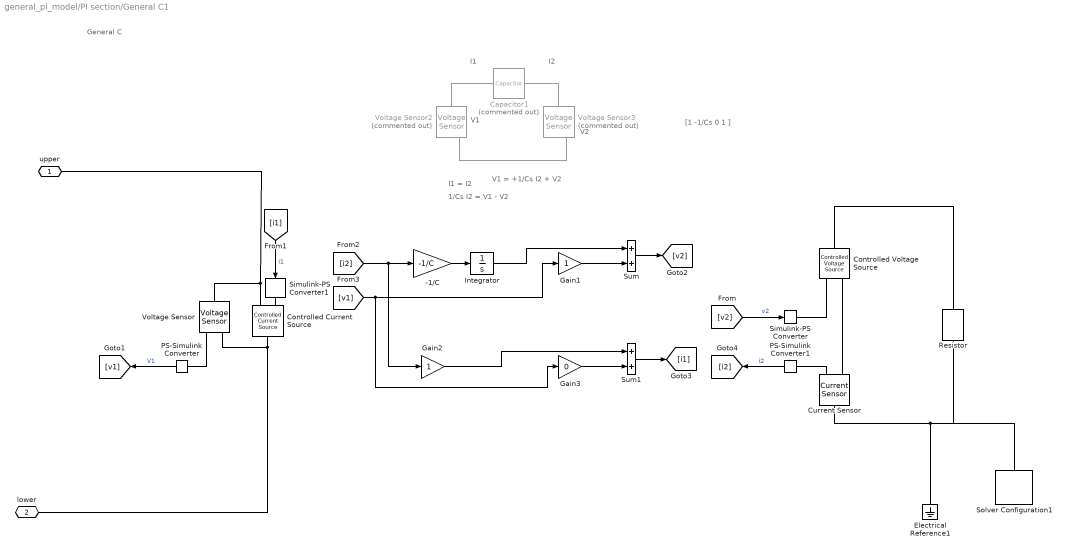
== system general_pi_model/PI section/General C1 ==
  note: General C
  note: V1
  note: V1 = +1/Cs I2 + V2
  note: I2
  note: I1 = I2
  note: 1/Cs I2 = V1 - V2
  note: V2
  note: [1 -1/Cs
      | 0 1 ]
  note: I1
  -1/C : Gain  Gain=-1/C
  Capacitor1 : fl_lib/Electrical/Electrical Elements/Capacitor  Commented=on  c=1e-6 F  r=1e-6 Ohm  g=0 1/Ohm  i_specify=off  i_priority=None  i=0 A  i_nominal_specify=off  i_nominal_value=1  i_nominal_unit=A  v_specify=off  v_priority=None  v=0 V  v_nominal_specify=off  v_nominal_value=1  v_nominal_unit=V  vc_specify=off  vc_priority=High  vc=0 V  vc_nominal_specify=off  vc_nominal_value=1  vc_nominal_unit=V
  Controlled Current Source : fl_lib/Electrical/Electrical Sources/Controlled Current Source
  Controlled Voltage Source : fl_lib/Electrical/Electrical Sources/Controlled Voltage Source
  Current Sensor : fl_lib/Electrical/Electrical Sensors/Current Sensor
  Electrical Reference1 : fl_lib/Electrical/Electrical Elements/Electrical Reference
  Gain1 : Gain
  Gain2 : Gain
  Gain3 : Gain  Gain=0
  Integrator : Integrator
  PS-Simulink Converter : nesl_utility/PS-Simulink Converter  PhysicalDomain=network_engine_domain  SubClassName=ps_output  LeftPortType=input  RightPortType=output  PseudoPeriodic=off  Frequencies=[]  VectorFormat=inherit  Unit=inherit  AffineConversion=off
  PS-Simulink Converter1 : nesl_utility/PS-Simulink Converter  PhysicalDomain=network_engine_domain  SubClassName=ps_output  LeftPortType=input  RightPortType=output  PseudoPeriodic=off  Frequencies=[]  VectorFormat=inherit  Unit=inherit  AffineConversion=off
  Resistor : fl_lib/Electrical/Electrical Elements/Resistor  R=1e-12 Ohm  i_specify=off  i_priority=None  i=0 A  i_nominal_specify=off  i_nominal_value=1  i_nominal_unit=A  v_specify=off  v_priority=None  v=0 V  v_nominal_specify=off  v_nominal_value=1  v_nominal_unit=V
  Simulink-PS Converter : nesl_utility/Simulink-PS Converter  PhysicalDomain=network_engine_domain  SubClassName=ps_input  LeftPortType=input  RightPortType=output  PseudoPeriodic=off  Frequencies=[]  NoiseDistribution=none  NoiseParameters=[]  Unit=V  AffineConversion=off  FilteringAndDerivatives=provide  SimscapeFilterOrder=1  InputFilterTimeConstant=0.001  UdotUserProvided=0
  Simulink-PS Converter1 : nesl_utility/Simulink-PS Converter  PhysicalDomain=network_engine_domain  SubClassName=ps_input  LeftPortType=input  RightPortType=output  PseudoPeriodic=off  Frequencies=[]  NoiseDistribution=none  NoiseParameters=[]  Unit=A  AffineConversion=off  FilteringAndDerivatives=provide  SimscapeFilterOrder=1  InputFilterTimeConstant=0.001  UdotUserProvided=0
  Solver Configuration1 : nesl_utility/Solver Configuration  PhysicalDomain=network_engine_domain  SubClassName=solver  LeftPortType=input  RightPortType=generic  Tones=[]  Harmonics=[]  SimulateNoise=off  Profile=off  UseLocalSampling=off  EnableSwitchedLinearOptims=on  FrequencyDomain=off  UseCCode=off  RelTol=0.001  AbsTol=0.001  MinStep=1e-09  ToWorkspace=off  RevertToSquareIcSolve=off  NumHomotopyIterations=100  PhasorMode=off  PhasorModeNumHarmonics=1  ConsistencySolver=NEWTON_XTOL_AFTER_FTOL  IndexReductionMethod=DerivativeReplacement  DoDC=off  ResidualTolerance=1e-09  ConsistencyTolSource=GLOBAL  ConsistencyAbsTol=0.001  ConsistencyRelTol=0.001  ConsistencyTolFactor=0.001  UseLocalSolver=off  LocalSolverChoice=NE_BACKWARD_EULER_ADVANCER  ResolveIndetEquations=on  FunctionEvalNumThread=1  LocalSolverSampleTime=0.001  DoFixedCost=off  MaxNonlinIter=3  MaxModeIter=2  ComputeImpulses=off  ImpulseIterations=2  LinearAlgebra=auto  LinearAlgebraNumThread=0  EquationFormulation=NE_TIME_EF  DelaysMemoryBudget=1024  AutomaticFiltering=on  FilteringTimeConstant=0.001  PartitionStorageMethod=AS_NEEDED  PartitionMemoryBudget=1024  PartitionMethod=ROBUST  MultibodyUseLocalSolver=off  MultibodyLocalSolverChoice=ODE1  MultibodyLocalSolverSampleTime=0.001
  Sum : Sum
  Sum1 : Sum
  Voltage Sensor : fl_lib/Electrical/Electrical Sensors/Voltage Sensor
  Voltage Sensor2 : fl_lib/Electrical/Electrical Sensors/Voltage Sensor  Commented=on
  Voltage Sensor3 : fl_lib/Electrical/Electrical Sensors/Voltage Sensor  Commented=on
  upper : PMIOPort  Side=Left
  lower : PMIOPort  Port=2  Side=Right
  wires:
  Sum1/1 -> [i1]
  Sum/1 -> [v2]
  [i2] -> Gain2/1, -1/C/1
  [v1] -> Gain1/1, Gain3/1
  Gain2/1 -> Sum1/1
  Gain3/1 -> Sum1/2
  Integrator/1 -> Sum/1
  Gain1/1 -> Sum/2
  -1/C/1 -> Integrator/1
  [i1] -> Simulink-PS Converter1/1  "i1"
  PS-Simulink Converter/1 -> [v1]  "V1"
  [v2] -> Simulink-PS Converter/1  "v2"
  PS-Simulink Converter1/1 -> [i2]  "i2"
  connections:
  Controlled Current Source/LConn1 -- lower/RConn1 -- Voltage Sensor/RConn2
  Voltage Sensor3/RConn2 -- Voltage Sensor2/RConn2
  Voltage Sensor3/LConn1 -- Capacitor1/RConn1
  Voltage Sensor2/LConn1 -- Capacitor1/LConn1
  Electrical Reference1/LConn1 -- Solver Configuration1/RConn1 -- Resistor/RConn1 -- Current Sensor/LConn1
  Resistor/LConn1 -- Controlled Voltage Source/LConn1
  Simulink-PS Converter/RConn1 -- Controlled Voltage Source/RConn1
  PS-Simulink Converter1/LConn1 -- Current Sensor/RConn1
  Voltage Sensor/RConn1 -- PS-Simulink Converter/LConn1
  Current Sensor/RConn2 -- Controlled Voltage Source/RConn2
  Controlled Current Source/RConn1 -- Simulink-PS Converter1/RConn1
  Controlled Current Source/RConn2 -- upper/RConn1 -- Voltage Sensor/LConn1

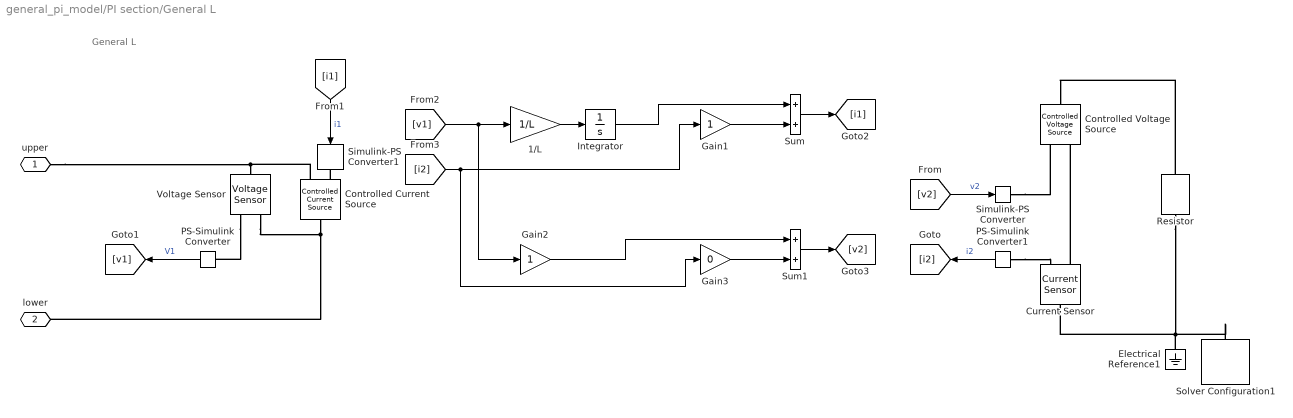
== system general_pi_model/PI section/General L ==
  note: General L
  1/L : Gain  Gain=1/L
  Controlled Current Source : fl_lib/Electrical/Electrical Sources/Controlled Current Source
  Controlled Voltage Source : fl_lib/Electrical/Electrical Sources/Controlled Voltage Source
  Current Sensor : fl_lib/Electrical/Electrical Sensors/Current Sensor
  Electrical Reference1 : fl_lib/Electrical/Electrical Elements/Electrical Reference
  Gain1 : Gain
  Gain2 : Gain
  Gain3 : Gain  Gain=0
  Integrator : Integrator
  PS-Simulink Converter : nesl_utility/PS-Simulink Converter  PhysicalDomain=network_engine_domain  SubClassName=ps_output  LeftPortType=input  RightPortType=output  PseudoPeriodic=off  Frequencies=[]  VectorFormat=inherit  Unit=inherit  AffineConversion=off
  PS-Simulink Converter1 : nesl_utility/PS-Simulink Converter  PhysicalDomain=network_engine_domain  SubClassName=ps_output  LeftPortType=input  RightPortType=output  PseudoPeriodic=off  Frequencies=[]  VectorFormat=inherit  Unit=inherit  AffineConversion=off
  Resistor : fl_lib/Electrical/Electrical Elements/Resistor  R=1e12 Ohm  i_specify=off  i_priority=None  i=0 A  i_nominal_specify=off  i_nominal_value=1  i_nominal_unit=A  v_specify=off  v_priority=None  v=0 V  v_nominal_specify=off  v_nominal_value=1  v_nominal_unit=V
  Simulink-PS Converter : nesl_utility/Simulink-PS Converter  PhysicalDomain=network_engine_domain  SubClassName=ps_input  LeftPortType=input  RightPortType=output  PseudoPeriodic=off  Frequencies=[]  NoiseDistribution=none  NoiseParameters=[]  Unit=V  AffineConversion=off  FilteringAndDerivatives=provide  SimscapeFilterOrder=1  InputFilterTimeConstant=0.001  UdotUserProvided=0
  Simulink-PS Converter1 : nesl_utility/Simulink-PS Converter  PhysicalDomain=network_engine_domain  SubClassName=ps_input  LeftPortType=input  RightPortType=output  PseudoPeriodic=off  Frequencies=[]  NoiseDistribution=none  NoiseParameters=[]  Unit=A  AffineConversion=off  FilteringAndDerivatives=provide  SimscapeFilterOrder=1  InputFilterTimeConstant=0.001  UdotUserProvided=0
  Solver Configuration1 : nesl_utility/Solver Configuration  PhysicalDomain=network_engine_domain  SubClassName=solver  LeftPortType=input  RightPortType=generic  Tones=[]  Harmonics=[]  SimulateNoise=off  Profile=off  UseLocalSampling=off  EnableSwitchedLinearOptims=on  FrequencyDomain=off  UseCCode=off  RelTol=0.001  AbsTol=0.001  MinStep=1e-09  ToWorkspace=off  RevertToSquareIcSolve=off  NumHomotopyIterations=100  PhasorMode=off  PhasorModeNumHarmonics=1  ConsistencySolver=NEWTON_XTOL_AFTER_FTOL  IndexReductionMethod=DerivativeReplacement  DoDC=off  ResidualTolerance=1e-09  ConsistencyTolSource=GLOBAL  ConsistencyAbsTol=0.001  ConsistencyRelTol=0.001  ConsistencyTolFactor=0.001  UseLocalSolver=off  LocalSolverChoice=NE_BACKWARD_EULER_ADVANCER  ResolveIndetEquations=on  FunctionEvalNumThread=1  LocalSolverSampleTime=0.001  DoFixedCost=off  MaxNonlinIter=3  MaxModeIter=2  ComputeImpulses=off  ImpulseIterations=2  LinearAlgebra=auto  LinearAlgebraNumThread=0  EquationFormulation=NE_TIME_EF  DelaysMemoryBudget=1024  AutomaticFiltering=on  FilteringTimeConstant=0.001  PartitionStorageMethod=AS_NEEDED  PartitionMemoryBudget=1024  PartitionMethod=ROBUST  MultibodyUseLocalSolver=off  MultibodyLocalSolverChoice=ODE1  MultibodyLocalSolverSampleTime=0.001
  Sum : Sum
  Sum1 : Sum
  Voltage Sensor : fl_lib/Electrical/Electrical Sensors/Voltage Sensor
  upper : PMIOPort  Side=Left
  lower : PMIOPort  Port=2  Side=Right
  wires:
  Sum1/1 -> [v2]
  Sum/1 -> [i1]
  [v1] -> Gain2/1, 1/L/1
  [i2] -> Gain1/1, Gain3/1
  Gain2/1 -> Sum1/1
  Gain3/1 -> Sum1/2
  Integrator/1 -> Sum/1
  Gain1/1 -> Sum/2
  1/L/1 -> Integrator/1
  [i1] -> Simulink-PS Converter1/1  "i1"
  PS-Simulink Converter/1 -> [v1]  "V1"
  [v2] -> Simulink-PS Converter/1  "v2"
  PS-Simulink Converter1/1 -> [i2]  "i2"
  connections:
  Controlled Current Source/LConn1 -- Voltage Sensor/RConn2 -- lower/RConn1
  Resistor/RConn1 -- Solver Configuration1/RConn1 -- Electrical Reference1/LConn1 -- Current Sensor/LConn1
  Resistor/LConn1 -- Controlled Voltage Source/LConn1
  Simulink-PS Converter/RConn1 -- Controlled Voltage Source/RConn1
  PS-Simulink Converter1/LConn1 -- Current Sensor/RConn1
  Voltage Sensor/RConn1 -- PS-Simulink Converter/LConn1
  Current Sensor/RConn2 -- Controlled Voltage Source/RConn2
  Controlled Current Source/RConn1 -- Simulink-PS Converter1/RConn1
  Controlled Current Source/RConn2 -- Voltage Sensor/LConn1 -- upper/RConn1

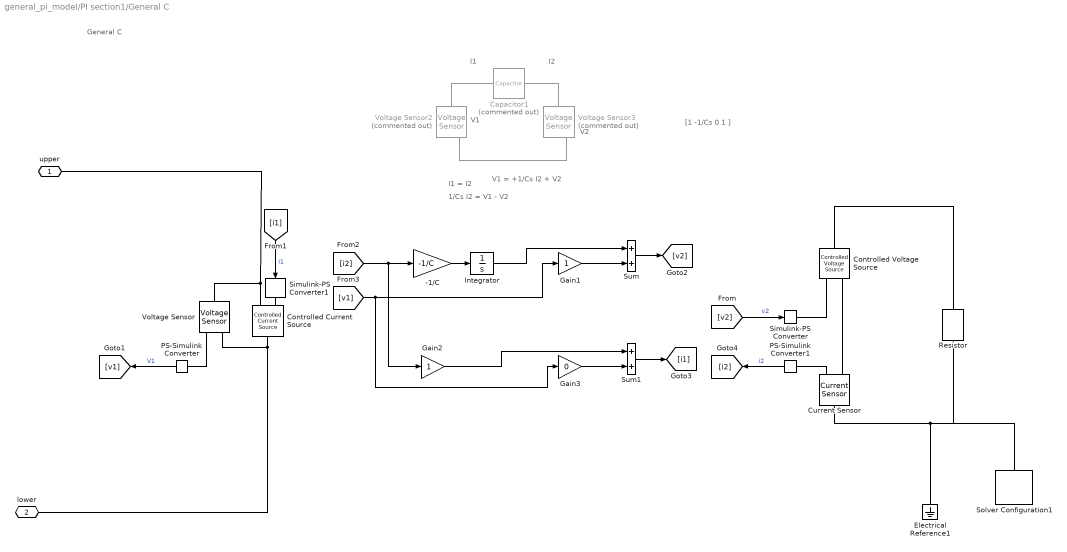
== system general_pi_model/PI section1/General C ==
  note: General C
  note: V1
  note: V1 = +1/Cs I2 + V2
  note: I2
  note: I1 = I2
  note: 1/Cs I2 = V1 - V2
  note: V2
  note: [1 -1/Cs
      | 0 1 ]
  note: I1
  -1/C : Gain  Gain=-1/C
  Capacitor1 : fl_lib/Electrical/Electrical Elements/Capacitor  Commented=on  c=1e-6 F  r=1e-6 Ohm  g=0 1/Ohm  i_specify=off  i_priority=None  i=0 A  i_nominal_specify=off  i_nominal_value=1  i_nominal_unit=A  v_specify=off  v_priority=None  v=0 V  v_nominal_specify=off  v_nominal_value=1  v_nominal_unit=V  vc_specify=off  vc_priority=High  vc=0 V  vc_nominal_specify=off  vc_nominal_value=1  vc_nominal_unit=V
  Controlled Current Source : fl_lib/Electrical/Electrical Sources/Controlled Current Source
  Controlled Voltage Source : fl_lib/Electrical/Electrical Sources/Controlled Voltage Source
  Current Sensor : fl_lib/Electrical/Electrical Sensors/Current Sensor
  Electrical Reference1 : fl_lib/Electrical/Electrical Elements/Electrical Reference
  Gain1 : Gain
  Gain2 : Gain
  Gain3 : Gain  Gain=0
  Integrator : Integrator
  PS-Simulink Converter : nesl_utility/PS-Simulink Converter  PhysicalDomain=network_engine_domain  SubClassName=ps_output  LeftPortType=input  RightPortType=output  PseudoPeriodic=off  Frequencies=[]  VectorFormat=inherit  Unit=inherit  AffineConversion=off
  PS-Simulink Converter1 : nesl_utility/PS-Simulink Converter  PhysicalDomain=network_engine_domain  SubClassName=ps_output  LeftPortType=input  RightPortType=output  PseudoPeriodic=off  Frequencies=[]  VectorFormat=inherit  Unit=inherit  AffineConversion=off
  Resistor : fl_lib/Electrical/Electrical Elements/Resistor  R=1e-12 Ohm  i_specify=off  i_priority=None  i=0 A  i_nominal_specify=off  i_nominal_value=1  i_nominal_unit=A  v_specify=off  v_priority=None  v=0 V  v_nominal_specify=off  v_nominal_value=1  v_nominal_unit=V
  Simulink-PS Converter : nesl_utility/Simulink-PS Converter  PhysicalDomain=network_engine_domain  SubClassName=ps_input  LeftPortType=input  RightPortType=output  PseudoPeriodic=off  Frequencies=[]  NoiseDistribution=none  NoiseParameters=[]  Unit=V  AffineConversion=off  FilteringAndDerivatives=provide  SimscapeFilterOrder=1  InputFilterTimeConstant=0.001  UdotUserProvided=0
  Simulink-PS Converter1 : nesl_utility/Simulink-PS Converter  PhysicalDomain=network_engine_domain  SubClassName=ps_input  LeftPortType=input  RightPortType=output  PseudoPeriodic=off  Frequencies=[]  NoiseDistribution=none  NoiseParameters=[]  Unit=A  AffineConversion=off  FilteringAndDerivatives=provide  SimscapeFilterOrder=1  InputFilterTimeConstant=0.001  UdotUserProvided=0
  Solver Configuration1 : nesl_utility/Solver Configuration  PhysicalDomain=network_engine_domain  SubClassName=solver  LeftPortType=input  RightPortType=generic  Tones=[]  Harmonics=[]  SimulateNoise=off  Profile=off  UseLocalSampling=off  EnableSwitchedLinearOptims=on  FrequencyDomain=off  UseCCode=off  RelTol=0.001  AbsTol=0.001  MinStep=1e-09  ToWorkspace=off  RevertToSquareIcSolve=off  NumHomotopyIterations=100  PhasorMode=off  PhasorModeNumHarmonics=1  ConsistencySolver=NEWTON_XTOL_AFTER_FTOL  IndexReductionMethod=DerivativeReplacement  DoDC=off  ResidualTolerance=1e-09  ConsistencyTolSource=GLOBAL  ConsistencyAbsTol=0.001  ConsistencyRelTol=0.001  ConsistencyTolFactor=0.001  UseLocalSolver=off  LocalSolverChoice=NE_BACKWARD_EULER_ADVANCER  ResolveIndetEquations=on  FunctionEvalNumThread=1  LocalSolverSampleTime=0.001  DoFixedCost=off  MaxNonlinIter=3  MaxModeIter=2  ComputeImpulses=off  ImpulseIterations=2  LinearAlgebra=auto  LinearAlgebraNumThread=0  EquationFormulation=NE_TIME_EF  DelaysMemoryBudget=1024  AutomaticFiltering=on  FilteringTimeConstant=0.001  PartitionStorageMethod=AS_NEEDED  PartitionMemoryBudget=1024  PartitionMethod=ROBUST  MultibodyUseLocalSolver=off  MultibodyLocalSolverChoice=ODE1  MultibodyLocalSolverSampleTime=0.001
  Sum : Sum
  Sum1 : Sum
  Voltage Sensor : fl_lib/Electrical/Electrical Sensors/Voltage Sensor
  Voltage Sensor2 : fl_lib/Electrical/Electrical Sensors/Voltage Sensor  Commented=on
  Voltage Sensor3 : fl_lib/Electrical/Electrical Sensors/Voltage Sensor  Commented=on
  upper : PMIOPort  Side=Left
  lower : PMIOPort  Port=2  Side=Right
  wires:
  Sum1/1 -> [i1]
  Sum/1 -> [v2]
  [i2] -> Gain2/1, -1/C/1
  [v1] -> Gain1/1, Gain3/1
  Gain2/1 -> Sum1/1
  Gain3/1 -> Sum1/2
  Integrator/1 -> Sum/1
  Gain1/1 -> Sum/2
  -1/C/1 -> Integrator/1
  [i1] -> Simulink-PS Converter1/1  "i1"
  PS-Simulink Converter/1 -> [v1]  "V1"
  [v2] -> Simulink-PS Converter/1  "v2"
  PS-Simulink Converter1/1 -> [i2]  "i2"
  connections:
  Controlled Current Source/LConn1 -- lower/RConn1 -- Voltage Sensor/RConn2
  Voltage Sensor3/RConn2 -- Voltage Sensor2/RConn2
  Voltage Sensor3/LConn1 -- Capacitor1/RConn1
  Voltage Sensor2/LConn1 -- Capacitor1/LConn1
  Electrical Reference1/LConn1 -- Solver Configuration1/RConn1 -- Resistor/RConn1 -- Current Sensor/LConn1
  Resistor/LConn1 -- Controlled Voltage Source/LConn1
  Simulink-PS Converter/RConn1 -- Controlled Voltage Source/RConn1
  PS-Simulink Converter1/LConn1 -- Current Sensor/RConn1
  Voltage Sensor/RConn1 -- PS-Simulink Converter/LConn1
  Current Sensor/RConn2 -- Controlled Voltage Source/RConn2
  Controlled Current Source/RConn1 -- Simulink-PS Converter1/RConn1
  Controlled Current Source/RConn2 -- upper/RConn1 -- Voltage Sensor/LConn1

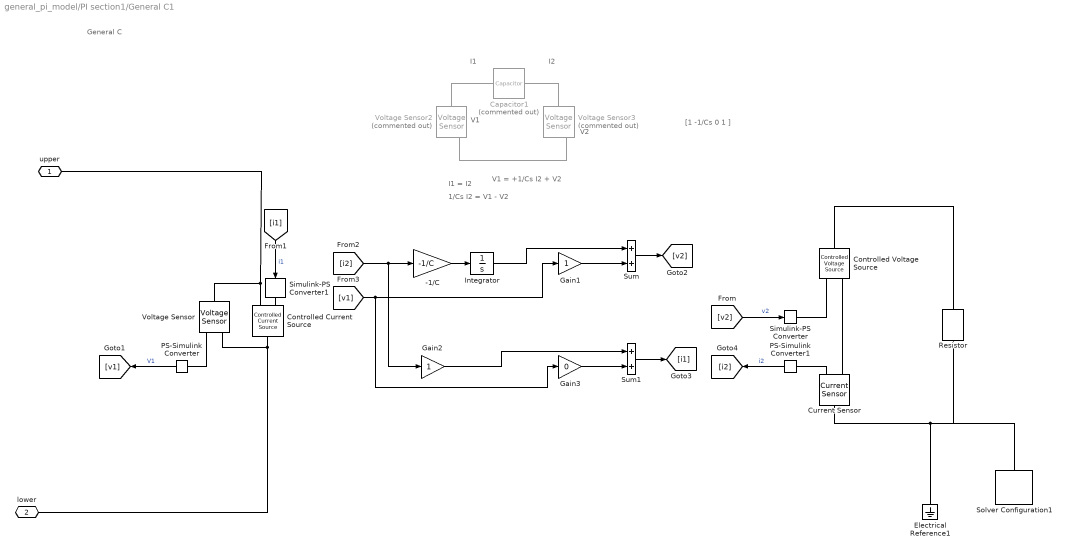
== system general_pi_model/PI section1/General C1 ==
  note: General C
  note: V1
  note: V1 = +1/Cs I2 + V2
  note: I2
  note: I1 = I2
  note: 1/Cs I2 = V1 - V2
  note: V2
  note: [1 -1/Cs
      | 0 1 ]
  note: I1
  -1/C : Gain  Gain=-1/C
  Capacitor1 : fl_lib/Electrical/Electrical Elements/Capacitor  Commented=on  c=1e-6 F  r=1e-6 Ohm  g=0 1/Ohm  i_specify=off  i_priority=None  i=0 A  i_nominal_specify=off  i_nominal_value=1  i_nominal_unit=A  v_specify=off  v_priority=None  v=0 V  v_nominal_specify=off  v_nominal_value=1  v_nominal_unit=V  vc_specify=off  vc_priority=High  vc=0 V  vc_nominal_specify=off  vc_nominal_value=1  vc_nominal_unit=V
  Controlled Current Source : fl_lib/Electrical/Electrical Sources/Controlled Current Source
  Controlled Voltage Source : fl_lib/Electrical/Electrical Sources/Controlled Voltage Source
  Current Sensor : fl_lib/Electrical/Electrical Sensors/Current Sensor
  Electrical Reference1 : fl_lib/Electrical/Electrical Elements/Electrical Reference
  Gain1 : Gain
  Gain2 : Gain
  Gain3 : Gain  Gain=0
  Integrator : Integrator
  PS-Simulink Converter : nesl_utility/PS-Simulink Converter  PhysicalDomain=network_engine_domain  SubClassName=ps_output  LeftPortType=input  RightPortType=output  PseudoPeriodic=off  Frequencies=[]  VectorFormat=inherit  Unit=inherit  AffineConversion=off
  PS-Simulink Converter1 : nesl_utility/PS-Simulink Converter  PhysicalDomain=network_engine_domain  SubClassName=ps_output  LeftPortType=input  RightPortType=output  PseudoPeriodic=off  Frequencies=[]  VectorFormat=inherit  Unit=inherit  AffineConversion=off
  Resistor : fl_lib/Electrical/Electrical Elements/Resistor  R=1e-12 Ohm  i_specify=off  i_priority=None  i=0 A  i_nominal_specify=off  i_nominal_value=1  i_nominal_unit=A  v_specify=off  v_priority=None  v=0 V  v_nominal_specify=off  v_nominal_value=1  v_nominal_unit=V
  Simulink-PS Converter : nesl_utility/Simulink-PS Converter  PhysicalDomain=network_engine_domain  SubClassName=ps_input  LeftPortType=input  RightPortType=output  PseudoPeriodic=off  Frequencies=[]  NoiseDistribution=none  NoiseParameters=[]  Unit=V  AffineConversion=off  FilteringAndDerivatives=provide  SimscapeFilterOrder=1  InputFilterTimeConstant=0.001  UdotUserProvided=0
  Simulink-PS Converter1 : nesl_utility/Simulink-PS Converter  PhysicalDomain=network_engine_domain  SubClassName=ps_input  LeftPortType=input  RightPortType=output  PseudoPeriodic=off  Frequencies=[]  NoiseDistribution=none  NoiseParameters=[]  Unit=A  AffineConversion=off  FilteringAndDerivatives=provide  SimscapeFilterOrder=1  InputFilterTimeConstant=0.001  UdotUserProvided=0
  Solver Configuration1 : nesl_utility/Solver Configuration  PhysicalDomain=network_engine_domain  SubClassName=solver  LeftPortType=input  RightPortType=generic  Tones=[]  Harmonics=[]  SimulateNoise=off  Profile=off  UseLocalSampling=off  EnableSwitchedLinearOptims=on  FrequencyDomain=off  UseCCode=off  RelTol=0.001  AbsTol=0.001  MinStep=1e-09  ToWorkspace=off  RevertToSquareIcSolve=off  NumHomotopyIterations=100  PhasorMode=off  PhasorModeNumHarmonics=1  ConsistencySolver=NEWTON_XTOL_AFTER_FTOL  IndexReductionMethod=DerivativeReplacement  DoDC=off  ResidualTolerance=1e-09  ConsistencyTolSource=GLOBAL  ConsistencyAbsTol=0.001  ConsistencyRelTol=0.001  ConsistencyTolFactor=0.001  UseLocalSolver=off  LocalSolverChoice=NE_BACKWARD_EULER_ADVANCER  ResolveIndetEquations=on  FunctionEvalNumThread=1  LocalSolverSampleTime=0.001  DoFixedCost=off  MaxNonlinIter=3  MaxModeIter=2  ComputeImpulses=off  ImpulseIterations=2  LinearAlgebra=auto  LinearAlgebraNumThread=0  EquationFormulation=NE_TIME_EF  DelaysMemoryBudget=1024  AutomaticFiltering=on  FilteringTimeConstant=0.001  PartitionStorageMethod=AS_NEEDED  PartitionMemoryBudget=1024  PartitionMethod=ROBUST  MultibodyUseLocalSolver=off  MultibodyLocalSolverChoice=ODE1  MultibodyLocalSolverSampleTime=0.001
  Sum : Sum
  Sum1 : Sum
  Voltage Sensor : fl_lib/Electrical/Electrical Sensors/Voltage Sensor
  Voltage Sensor2 : fl_lib/Electrical/Electrical Sensors/Voltage Sensor  Commented=on
  Voltage Sensor3 : fl_lib/Electrical/Electrical Sensors/Voltage Sensor  Commented=on
  upper : PMIOPort  Side=Left
  lower : PMIOPort  Port=2  Side=Right
  wires:
  Sum1/1 -> [i1]
  Sum/1 -> [v2]
  [i2] -> Gain2/1, -1/C/1
  [v1] -> Gain1/1, Gain3/1
  Gain2/1 -> Sum1/1
  Gain3/1 -> Sum1/2
  Integrator/1 -> Sum/1
  Gain1/1 -> Sum/2
  -1/C/1 -> Integrator/1
  [i1] -> Simulink-PS Converter1/1  "i1"
  PS-Simulink Converter/1 -> [v1]  "V1"
  [v2] -> Simulink-PS Converter/1  "v2"
  PS-Simulink Converter1/1 -> [i2]  "i2"
  connections:
  Controlled Current Source/LConn1 -- lower/RConn1 -- Voltage Sensor/RConn2
  Voltage Sensor3/RConn2 -- Voltage Sensor2/RConn2
  Voltage Sensor3/LConn1 -- Capacitor1/RConn1
  Voltage Sensor2/LConn1 -- Capacitor1/LConn1
  Electrical Reference1/LConn1 -- Solver Configuration1/RConn1 -- Resistor/RConn1 -- Current Sensor/LConn1
  Resistor/LConn1 -- Controlled Voltage Source/LConn1
  Simulink-PS Converter/RConn1 -- Controlled Voltage Source/RConn1
  PS-Simulink Converter1/LConn1 -- Current Sensor/RConn1
  Voltage Sensor/RConn1 -- PS-Simulink Converter/LConn1
  Current Sensor/RConn2 -- Controlled Voltage Source/RConn2
  Controlled Current Source/RConn1 -- Simulink-PS Converter1/RConn1
  Controlled Current Source/RConn2 -- upper/RConn1 -- Voltage Sensor/LConn1
